simulink model "OverlapSaveFIR_11paths"  (R2024a)
settings: Solver=VariableStepAuto  StartTime=0.0  StopTime=8192  RelTol=1e-3
InitFcn:
  | N=256;
  | h=firpm(128,[0;0.4;0.5;1],[1;1;0;0],[1;50],{20});
  | hc=fft(h,N);
  | h_quant = int16(2^14*hc/max(hc));
  | M=length(h);
undefined symbols (not defined in the file): DUT, overlapSaveFIR_11paths, S, vsva2197, xcvc1902
libraries: aieBasic x44, aieUtilities x11, dspxfrm3 x2, dspsrcs4 x2, vmcUtilities x1
(part 1 of 2)
settings Model: Creator=catalinb  LastModifiedBy=sdegala
settings OptimizationCC: ReuseModelBlockBuffer=off
settings DebuggingCC: UnconnectedInputMsg=warning  UnconnectedOutputMsg=warning  UnconnectedLineMsg=warning
settings HardwareCC: ProdBitPerPointer=32  ProdBitPerSizeT=32  ProdBitPerPtrDiffT=32  ProdLargestAtomicFloat=None  ProdIntDivRoundTo=Undefined  ProdEndianess=Unspecified  ProdWordSize=32  ProdHWDeviceType=ASIC/FPGA->ASIC/FPGA  TargetBitPerLong=64  TargetBitPerPointer=64  TargetBitPerSizeT=64  TargetBitPerPtrDiffT=64  TargetLongLongMode=on  TargetIntDivRoundTo=Zero  TargetEndianess=LittleEndian  TargetWordSize=64  TargetHWDeviceType=Custom Processor->MATLAB Host Computer  ProdEqTarget=off
settings ModelReferenceCC: EnableRefExpFcnMdlSchedulingChecks=on
settings RTWCC: GPUComputeCapability=3.5  DLArmComputeVersion=19.05
settings ConfigComp: CovBoundaryAbsTol=1.0e-5

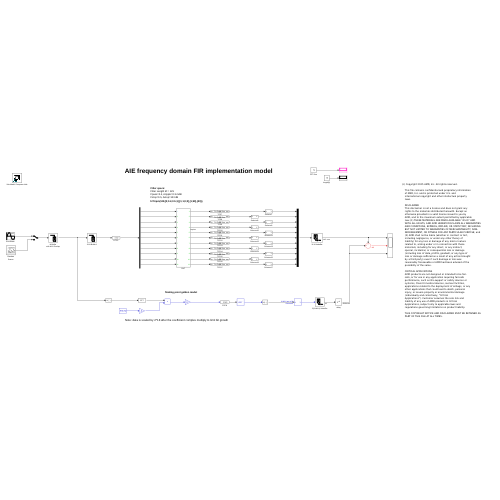
[thumbnail: Simulink's stored preview of the top-level diagram]
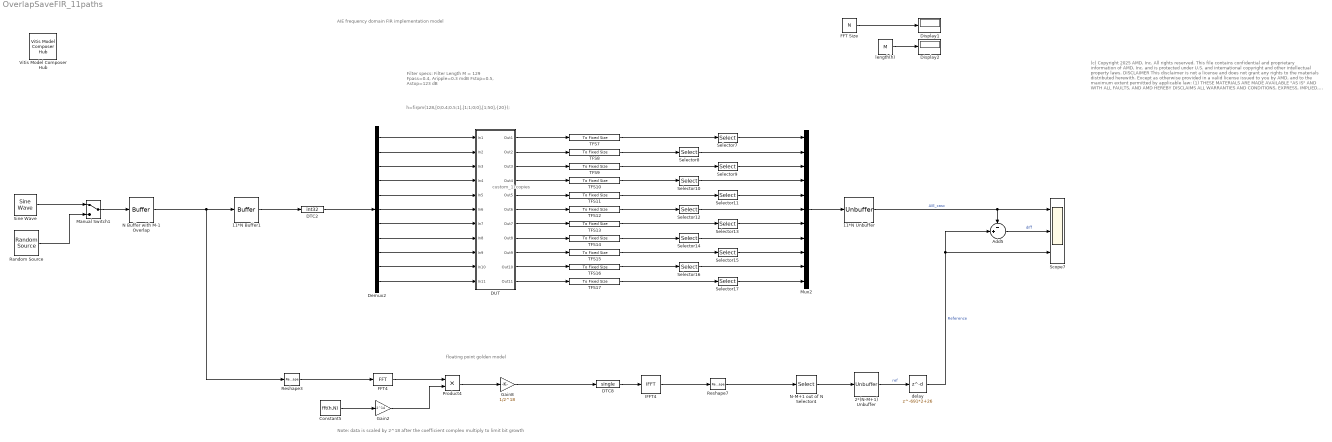
== system OverlapSaveFIR_11paths ==
  note: custom_11copies
  note: AIE frequency domain FIR implementation model
  note: floating point golden model
  note: Note: data is scaled by 2^18 after the coefficient complex multiply to limit bit growth
  note: h=firpm(128,[0;0.4;0.5;1],[1;1;0;0],[1;50],{20});
  note: Filter specs:
      | Filter Length M = 129
      | Fpass=0.4, Aripple=0.3 mdB
      | Fstop=0.5, Astop=123 dB
  note: (c) Copyright 2025 AMD, Inc. All rights reserved.
      |
      | This file contains confidential and proprietary information
      | of AMD, Inc. and is protected under U.S. and
      | international copyright and other intellectual property
      | laws.
      |
      | DISCLAIMER
      | This disclaimer is not a license and does not grant any
      | rights to the materials distributed herewith. Except as
      | otherwise provided in a valid license issued to you by
      | AMD, and to the maximum extent permitted by applicable
      | law: (1) THESE MATERIALS ARE MADE AVAILABLE "AS IS" AND
      | WITH ALL FAULTS, AND AMD HEREBY DISCLAIMS ALL WARRANTIES
      | AND CONDITIONS, EXPRESS, IMPLIED, OR STATUTORY, INCLUDING
      | BUT NOT LIMITED TO WARRANTIES OF MERCHANTABILITY, NON-
      | INFRINGEMENT, OR FITNESS FOR ANY PARTICULAR PURPOSE; and
      | (2) AMD shall not be liable (whether in contract or tort,
      | including negligence, or under any other theory of
      | liability) for any loss or damage of any kind or nature
      | related to, arising under or in connection with these
      | materials, including for any direct, or any indirect,
      | special, incidental, or consequential loss or damage
      | (including loss of data, profits, goodwill, or any type of
      | loss or damage suffered as a result of any action brought
      | by a third party) even if such damage or loss was
      | reasonably foreseeable or AMD had been advised of the
      | possibility of the same.
      |
      | CRITICAL APPLICATIONS
      | AMD products are not designed or intended to be fail-
      | safe, or for use in any application requiring fail-safe
      | performance, such as life-support or safety devices or
      | systems, Class III medical devices, nuclear facilities,
      | applications related to the deployment of airbags, or any
      | other applications that could lead to death, personal
      | injury, or severe property or environmental damage
      | (individually and collectively, "Critical
      | Applications"). Customer assumes the sole risk and
      | liability of any use of AMD products in Critical
      | Applications, subject only to applicable laws and
      | regulations governing limitations on product liability.
      |
      | THIS COPYRIGHT NOTICE AND DISCLAIMER MUST BE RETAINED AS
      | PART OF THIS FILE AT ALL TIMES.
  11*N Buffer1 : Buffer  N=11*N  OutputFrames=off
  11*N Unbuffer : Unbuffer
  2*(N-M+1) Unbuffer : Unbuffer
  Add5 : Sum  Inputs=-+|
  Constant5 : Constant  Value=fft(h,N)  SampleTime=2*(N-M+1)
  DTC2 : DataTypeConversion  OutDataTypeStr=int32  SaturateOnIntegerOverflow=off  RndMeth=Floor
  DTC8 : DataTypeConversion  OutDataTypeStr=single  SaturateOnIntegerOverflow=off  RndMeth=Floor
  DUT : Subsystem
  Demux2 : Demux  Outputs=11
  Display1 : Display
  Display2 : Display
  FFT Size : Constant  Value=N
  FFT4 : dspxfrm3/FFT  FFTImplementation=Auto  CompMethod=Table lookup  TableOpt=NEW  TableOptActive=Speed  BitRevOrder=off  Normalize=off  InheritFFTLength=on  FFTLength=64  WrapInput=on  roundingMode=Floor  overflowMode=off  firstCoeffDataTypeStr=Inherit: Same word length as input  firstCoeffLastDataTypeStr=Inherit: Same word length as input  outputMin=[]  outputMax=[]
  Gain2 : Gain  Gain=2^14  OutDataTypeStr=single
  Gain8 : Gain  Gain=1/2^18  OutDataTypeStr=single
  IFFT4 : dspxfrm3/IFFT  FFTImplementation=Auto  CompMethod=Table lookup  TableOpt=NEW  TableOptActive=Speed  BitRevOrder=off  cs_in=off  Normalize=off  InheritFFTLength=on  FFTLength=64  WrapInput=on  mode=Complex  outSamplingMode=Sample based  roundingMode=Floor  overflowMode=off  firstCoeffDataTypeStr=Inherit: Same word length as input  firstCoeffLastDataTypeStr=Inherit: Same word length as input  outputMin=[]  outputMax=[]
  Manual Switch1 : ManualSwitch
  Mux2 : Mux  Inputs=11
  N Buffer with M-1 Overlap : Buffer  N=N  V=M-1  OutputFrames=off
  N-M+1 out of N Selector4 : Selector  InputPortWidth=N  IndexOptions=Index vector (dialog)  Indices=[length(h):N]  OutputSizes=1
  Product4 : Product
  Random Source : dspsrcs4/Random Source  SrcType=Uniform  MinVal=-2^10  MaxVal=2^10  MeanVal=0  VarVal=1e-4  RepMode=Not repeatable  rawSeed=1  IsInherit=off  SampTime=0.5  SampFrame=256  OutComplex=Complex  DataType=single  SimulateUsing=Interpreted execution
  Reshape3 : Reshape
  Reshape7 : Reshape
  Scope7 : Scope  NumInputPorts=3
  Selector{7..17} (11 alike) : Selector  InputPortWidth=N  IndexOptions=Index vector (dialog)  Indices=[length(h):N]  OutputSizes=1
  Sine Wave : dspsrcs4/Sine Wave  Amplitude=2^10  Frequency=0.05  Phase=0  SampleMode=Discrete  OutComplex=Complex  CompMethod=Table lookup  TableSize=Speed  SampleTime=0.5  SamplesPerFrame=256  ResetState=Restart at time zero  OutputFrames=off  dataType=single  wordLen=32  udDataType=sfix(16)  fracBitsMode=User-defined  numFracBits=0  OutDataTypeStr=single  LastOutDataTypeStr=single
  TFS{7..17} (11 alike) : aieUtilities/To Fixed Size  Mode=Stop simulation when input variable-size signal is not full  OutputSize=Inherit: Same as input  CopyMethod=Buffer samples to form output  HasStatusOutput=on
  Vitis Model Composer Hub : vmcUtilities/Vitis Model Composer Hub  Tag=genX  CodeGeneration=off  SubsystemName=DUT  BlockHierPath=overlapSaveFIR_11paths/DUT  CompilationType=AIECompilation  SubsystemType=AIENode  ExportTypeV2=Graph Code  AIEArrayConfig=Use entire AIE array  StartColumn=1  NumberOfColumns=1  TargetDirectory=./code  exportDesign=on  analyzeDesign=off  validateDesignOnHw=off  ExportType=AI Engines  IpVendor=xilinx.com  IpLibrary=hls  IpVersion=1.0  IpHWLanguage=Verilog  AieCompilerOptions={'--xlopt=2', '--Xmapper=BufferOptLevel7'}  AieSimulatorOptions={}  CreateTestbench=off  TestbenchStackSize=10  RunRtlSim=off  RunCSim=off  RunAieSim=on  AieSimTimeout=50000  RunAieSimProfiling=off  LaunchVitisAnalyzer=on  PlotOutput=off  RunX86Sim=off  X86SimTimeout=10  GenHwImage=off  GenLibadfXo=off  GenHwValidationCode=off  PlatformType=Not Specified  HwSystemType=Baremetal  HwValidationTarget=hw  ProjDevice=Versal VCK190 Evaluation Platform with New SD Level Shifter (xcvc1902-vsva2197-2MP-e-S)  ProjDevicePart=xcvc1902-vsva2197-2MP-e-S  AIEType=AIE  SamplePeriod=-1  ClockFrequency=200  DataPathParallelism=1  xilinxfamily=versalaicore  part=xcvc1902  speed=-2MP-e-S  package=vsva2197  directory=./netlist  testbench=off  incr_netlist=off  synthesis_tool=Vivado  clock_wrapper=Clock Enables  dbl_ovrd=According to Block Masks  dcm_input_clock_period=10  sysclk_period=10  simulink_period=1  eval_field=0  IPInfoJsonString="{\"DUTSubsystemName\":\"DUT\",\"AIESubsystem\":{\"SubsystemName\":\"DUT\",\"TargetDirectory\":\"./code\",\"AIEArrayConfig\":\"Use entire AIE array\",\"StartColumn\":\"0\",\"NumberOfColumns\":\"1\"},\"SubsystemTag\":\"AIENode\"}"  LogFileName=/proj/xhdhdstaff5/sdegala/Head1/HEAD/2025_2_work/FDF/code/model_composer.log  NThreads=4  IPConfigFile=/tmp/vmctmp-10983784262153251499/overlapSaveFIR_11paths_ipconfig.json
  delay : Delay  DelayLength=691*2+26
  length(h) : Constant  Value=M
  wires:
  FFT Size/1 -> Display1/1
  length(h)/1 -> Display2/1
  N-M+1 out of N Selector4/1 -> 2*(N-M+1) Unbuffer/1
  Reshape7/1 -> N-M+1 out of N Selector4/1
  Reshape3/1 -> FFT4/1
  IFFT4/1 -> Reshape7/1
  Constant5/1 -> Gain2/1
  Gain2/1 -> Product4/2
  Product4/1 -> Gain8/1
  FFT4/1 -> Product4/1
  DTC8/1 -> IFFT4/1
  N Buffer with M-1 Overlap/1 -> 11*N Buffer1/1, Reshape3/1
  Gain8/1 -> DTC8/1
  DUT/4(Out4) -> TFS10/1
  TFS12/1 -> Selector12/1
  Demux2/7 -> DUT/7(In7)
  Mux2/1 -> 11*N Unbuffer/1
  Selector8/1 -> Mux2/2
  11*N Unbuffer/1 -> Scope7/1, Add5/1  "AIE_casc"
  Selector10/1 -> Mux2/4
  TFS8/1 -> Selector8/1
  Demux2/6 -> DUT/6(In6)
  DUT/6(Out6) -> TFS12/1
  DUT/5(Out5) -> TFS11/1
  TFS11/1 -> Selector11/1
  DUT/1(Out1) -> TFS7/1
  Demux2/2 -> DUT/2(In2)
  TFS9/1 -> Selector9/1
  Selector12/1 -> Mux2/6
  Demux2/3 -> DUT/3(In3)
  Selector9/1 -> Mux2/3
  TFS13/1 -> Selector13/1
  DUT/7(Out7) -> TFS13/1
  DUT/2(Out2) -> TFS8/1
  Selector11/1 -> Mux2/5
  Demux2/4 -> DUT/4(In4)
  Add5/1 -> Scope7/2  "diff"
  Selector13/1 -> Mux2/7
  Demux2/5 -> DUT/5(In5)
  TFS10/1 -> Selector10/1
  11*N Buffer1/1 -> DTC2/1
  DTC2/1 -> Demux2/1
  Demux2/1 -> DUT/1(In1)
  DUT/3(Out3) -> TFS9/1
  Selector7/1 -> Mux2/1
  TFS7/1 -> Selector7/1
  Demux2/8 -> DUT/8(In8)
  Demux2/9 -> DUT/9(In9)
  Demux2/10 -> DUT/10(In10)
  Demux2/11 -> DUT/11(In11)
  TFS14/1 -> Selector14/1
  Selector17/1 -> Mux2/11
  Selector15/1 -> Mux2/9
  DUT/11(Out11) -> TFS17/1
  Selector16/1 -> Mux2/10
  TFS15/1 -> Selector15/1
  DUT/9(Out9) -> TFS15/1
  DUT/10(Out10) -> TFS16/1
  Selector14/1 -> Mux2/8
  TFS16/1 -> Selector16/1
  DUT/8(Out8) -> TFS14/1
  TFS17/1 -> Selector17/1
  Sine Wave/1 -> Manual Switch1/1
  Manual Switch1/1 -> N Buffer with M-1 Overlap/1
  Random Source/1 -> Manual Switch1/2
  2*(N-M+1) Unbuffer/1 -> delay/1  "ref"
  delay/1 -> Scope7/3, Add5/2  "Reference"
